simulink model "FFDF"  (Simulink 7.9)
settings: Solver=ode45  StartTime=0.0  StopTime=10.0  RelTol=1e-3
values from neighbouring files (symbols this model uses):
  A1 = [-(Rg+Ron+Rp)/(Lm*(n^2))  -R/((R+Rc)*n*Lm); R/((R+Rc)*n*C)  -1/((R+Rc)*C)]    [ESR.m]    (also in b.m; c.m; d.m = [-(Ron+Rg+Rp)/(n^2*Lm) -R/(n*Lm*(R+Rc)); R/((R+Rc)*n*C) -1/(; g2.m = [-(Ron+Rg+Rp)/(n^2*Lm) -R/(n*Lm*(R+Rc)); R/((R+Rc)*n*C) -1/()
  A2 = [-Rp/(Lm*((n+1)^2))  -R/((n+1)*(R+Rc)*Lm); R/((n+1)*(R+Rc)*C)  -1/((R+Rc)*C)]    [ESR.m]    (also in b.m; c.m; d.m = [-Rp/((n+1)^2*Lm) -R/((n+1)*Lm*(R+Rc)); R/((n+1)*(R+Rc)*C) -; g2.m = [-Rp/((n+1)^2*Lm) -R/((n+1)*Lm*(R+Rc)); R/((n+1)*(R+Rc)*C) -)
  B1 = [1/(n*Lm)  -1/(n*Lm)  0  0 0; 0  0  0  0 0]    [ESR.m]    (also in b.m; c.m; d.m = [1/(n*Lm) -1/(n*Lm) 0 0; 0 0 0 0]; g2.m = [1/(n*Lm) -1/(n*Lm) 0 0; 0 0 0 0])
  B2 = [0  0  -1/((n+1)*Lm)  -1/(Lm*(n+1)) 0; 0  0  0  0 0]    [ESR.m]    (also in b.m; c.m; d.m = [0 0 -1/((n+1)*Lm) -1/((n+1)*Lm); 0 0 0 0]; g2.m = [0 0 -1/((n+1)*Lm) -1/((n+1)*Lm); 0 0 0 0])
settings Model: Creator=ghita  LastModifiedBy=ghita

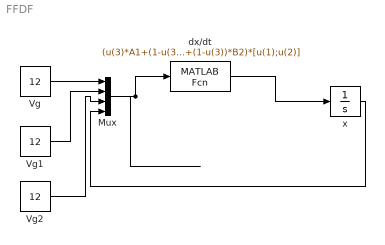
== system FFDF ==
  Mux : Mux
  Vg : Constant  Value=12
  Vg1 : Constant  Value=12
  Vg2 : Constant  Value=12
  dx/dt : MATLABFcn  MATLABFcn=(u(3)*A1+(1-u(3))*A2)*[u(4);u(5)]+(u(3)*B1+(1-u(3))*B2)*[u(1);u(2)]  OutputDimensions=2
  x : Integrator
  wires:
  Mux/1 -> dx/dt/1
  dx/dt/1 -> x/1
  Vg/1 -> Mux/1
  Vg1/1 -> Mux/2
  Vg2/1 -> Mux/3
  x/1 -> Mux/4
